simulink model "HILS_Px4"  (Simulink 8.6)
settings: Solver=FixedStepDiscrete  StartTime=0.0  StopTime=inf  FixedStep=0.01  RelTol=1e-3
PreLoadFcn:
  | addpath([cd filesep 'QuadCom']);
InitFcn:
  | %cd('..\Uart_Com');
undefined symbols (not defined in the file or in its folder): DiscIntNeverNeededParam
libraries: vrlib x1, sldrtlib x1
settings Model: Creator=Michael  LastModifiedBy=Xuan Mung  ExtModeTrigDuration=2
settings DataIOCC: SignalLoggingSaveFormat=Dataset
settings OptimizationCC: ExpressionDepthLimit=128  OptimizeModelRefInitCode=on  LifeSpan=1
settings DebuggingCC: SolverPrmCheckMsg=none  FcnCallInpInsideContextMsg=EnableAllAsError  StateNameClashWarn=none
settings HardwareCC: ProdBitPerInt=16  ProdBitPerPointer=8  ProdIntDivRoundTo=Zero  ProdEndianess=LittleEndian  ProdWordSize=8  ProdHWDeviceType=Atmel->AVR
settings RTWCC: SystemTargetFile=realtime.tlc  GenerateMakefile=off  TemplateMakefile=realtime.tmf  Description=Run on Target Hardware  RTWVerbose=off
settings STFCustomTargetCC: TargetLibSuffix=.a  GenerateSampleERTMain=on  ERTCustomFileBanners=on  SupportNonInlinedSFcns=off  SupportVariableSizeSignals=on  MATLABClassNameForMDSCustomization=Simulink.SoftwareTarget.ERTCustomization  GRTInterface=off  SystemTargetFile=realtime.tlc
settings ERTTargetCC: MultiwordLength=2048  GenerateSampleERTMain=on  ParMdlRefBuildCompliant=off  CompOptLevelCompliant=off  ConcurrentExecutionCompliant=off  CombineOutputUpdateFcns=off  ERTFirstTimeCompliant=off  SupportContinuousTime=on  SupportVariableSizeSignals=on  ModelStepFunctionPrototypeControlCompliant=off  CPPClassGenCompliant=off  UseToolchainInfoCompliant=off  ExtModeTransport=3  ExtModeMexFile=ext_serial_win32_comm_rtt  ExtModeMexArgs=0 1 9600  ERTSrcFileBannerTemplate=realtime_code_template.cgt  ERTHdrFileBannerTemplate=realtime_code_template.cgt  ERTDataSrcFileTemplate=realtime_code_template.cgt  ERTDataHdrFileTemplate=realtime_code_template.cgt  ERTCustomFileTemplate=realtime_file_process.tlc  ConvertIfToSwitch=off  SuppressUnreachableDefaultCases=off
settings ConfigComp: CovSFcnEnable=off
settings SettingsController: Description=Run on Hardware Dialog  TargetExtensionPlatform=None
settings MATStruct: Set_host_COM_port=[0.0]  COM_port_number=1  COM_port_baud_rate=115200  Enable_overrun_detection=[0.0]  Digital_output_to_set_on_overrun=13  Extmode_interface_arduino=[0.0]  Analog_input_reference_voltage=[0.0]  Serial0_baud_rate=9600  Serial1_baud_rate=9600  Serial2_baud_rate=9600  Serial3_baud_rate=9600  Local_ip_address=192.168.0.20  Local_mac_address=DE:AD:BE:EF:FE:ED  Wifi_ip_address=192.168.1.20  Wifi_SSID=yourNetwork  Set_Wifi_Encryption=[0.0]  Wifi_WEP_key=D0D0DEADF00DABBADEAFBEADED  Wifi_WEP_key_index=0  Wifi_WPA_password=secretPassword

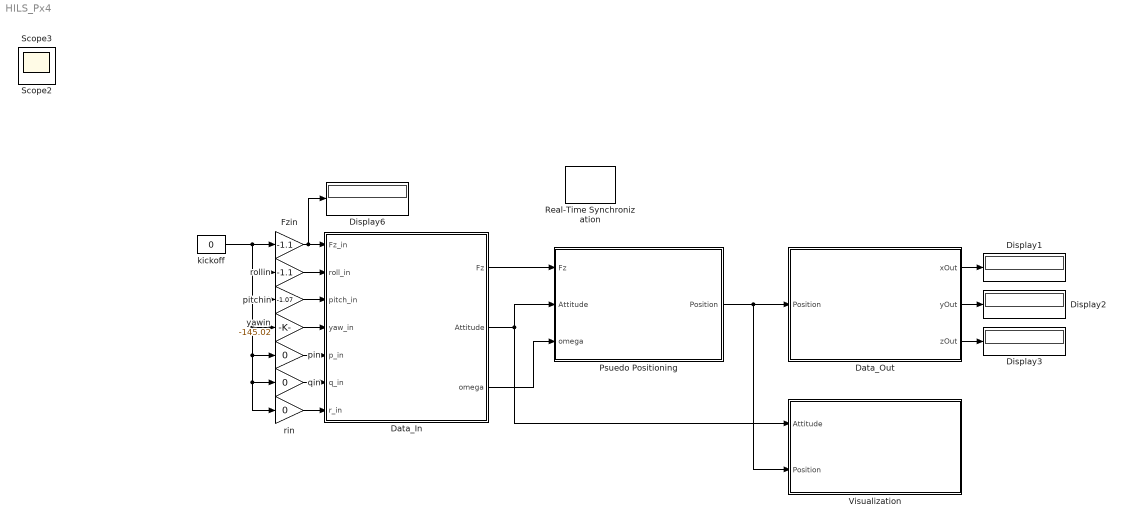
== system HILS_Px4 ==
  Data_In : Subsystem
  Data_Out : Subsystem
  Display{1..3,6} (4 alike) : Display
  Fzin : Gain  Gain=-1.1
  Psuedo Positioning : Subsystem
  Real-Time Synchronization : sldrtlib/Real-Time Synchronization  SampleTime=0.1  MaxMissedTicks=10  ShowMissedTicks=off  YieldWhenWaiting=off
  Visualization : Subsystem
  kickoff : Constant  Value=0
  pin : Gain  Gain=0
  pitchin : Gain  Gain=-1.07
  qin : Gain  Gain=0
  rin : Gain  Gain=0
  rollin : Gain  Gain=-1.1
  yawin : Gain  Gain=-145.02
  Scope2 : Scope
  Scope3 : Scope
  wires:
  Data_Out/1(xOut) -> Display1/1
  Data_Out/2(yOut) -> Display2/1
  Data_Out/3(zOut) -> Display3/1
  Fzin/1 -> Display6/1, Data_In/1(Fz_in)
  rollin/1 -> Data_In/2(roll_in)
  pitchin/1 -> Data_In/3(pitch_in)
  yawin/1 -> Data_In/4(yaw_in)
  pin/1 -> Data_In/5(p_in)
  qin/1 -> Data_In/6(q_in)
  rin/1 -> Data_In/7(r_in)
  kickoff/1 -> pitchin/1, yawin/1, pin/1, qin/1, rin/1, rollin/1, Fzin/1
  Data_In/1(Fz) -> Psuedo Positioning/1(Fz)
  Data_In/2(Attitude) -> Visualization/1(Attitude), Psuedo Positioning/2(Attitude)
  Data_In/3(omega) -> Psuedo Positioning/3(omega)
  Psuedo Positioning/1(Position) -> Visualization/2(Position), Data_Out/1(Position)

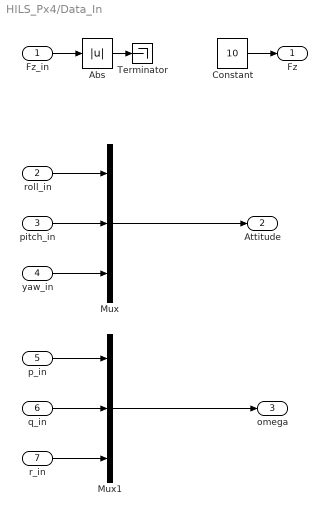
== system HILS_Px4/Data_In ==
  Fz_in : Inport
  roll_in : Inport  Port=2
  pitch_in : Inport  Port=3
  yaw_in : Inport  Port=4
  p_in : Inport  Port=5
  q_in : Inport  Port=6
  r_in : Inport  Port=7
  Abs : Abs
  Constant : Constant  Value=10
  Mux : Mux  Inputs=3
  Mux1 : Mux  Inputs=3
  Terminator : Terminator
  Fz : Outport
  Attitude : Outport  Port=2
  omega : Outport  Port=3
  wires:
  Mux/1 -> Attitude/1
  Mux1/1 -> omega/1
  roll_in/1 -> Mux/1
  pitch_in/1 -> Mux/2
  yaw_in/1 -> Mux/3
  p_in/1 -> Mux1/1
  q_in/1 -> Mux1/2
  r_in/1 -> Mux1/3
  Fz_in/1 -> Abs/1
  Constant/1 -> Fz/1
  Abs/1 -> Terminator/1

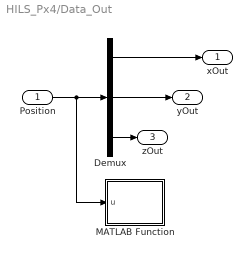
== system HILS_Px4/Data_Out ==
  Position : Inport
  Demux : Demux  Outputs=3
  MATLAB Function : MATLAB Function  TreatAsAtomicUnit=on
  xOut : Outport
  yOut : Outport  Port=2
  zOut : Outport  Port=3
  wires:
  Position/1 -> Demux/1, MATLAB Function/1(u)
  Demux/1 -> xOut/1
  Demux/2 -> yOut/1
  Demux/3 -> zOut/1

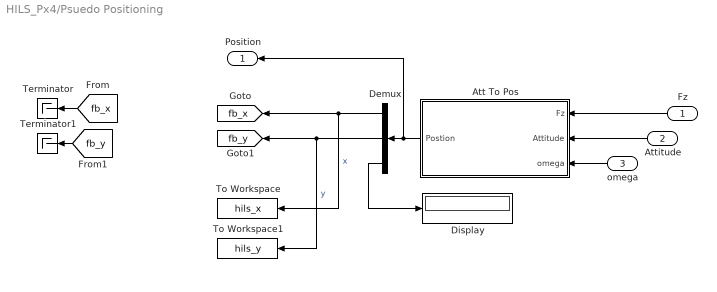
== system HILS_Px4/Psuedo Positioning ==
  Fz : Inport
  Attitude : Inport  Port=2
  omega : Inport  Port=3
  Att To Pos : Subsystem
  Demux : Demux  Outputs=3
  Display : Display
  Terminator : Terminator
  Terminator1 : Terminator
  To Workspace : ToWorkspace  VariableName=hils_x  SaveFormat=Timeseries  SampleTime=-1
  To Workspace1 : ToWorkspace  VariableName=hils_y  SaveFormat=Timeseries  SampleTime=-1
  Position : Outport
  tag scope: fb_x=global, fb_y=global
  wires:
  Attitude/1 -> Att To Pos/2(Attitude)
  Att To Pos/1(Postion) -> Position/1, Demux/1
  Demux/1 -> [fb_x], To Workspace/1  "x"
  Demux/2 -> [fb_y], To Workspace1/1  "y"
  omega/1 -> Att To Pos/3(omega)
  Demux/3 -> Display/1
  Fz/1 -> Att To Pos/1(Fz)
  [fb_x] -> Terminator/1
  [fb_y] -> Terminator1/1

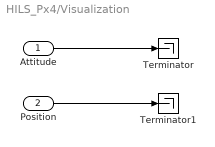
== system HILS_Px4/Visualization ==
  Attitude : Inport
  Position : Inport  Port=2
  Terminator : Terminator
  Terminator1 : Terminator
  wires:
  Attitude/1 -> Terminator/1
  Position/1 -> Terminator1/1

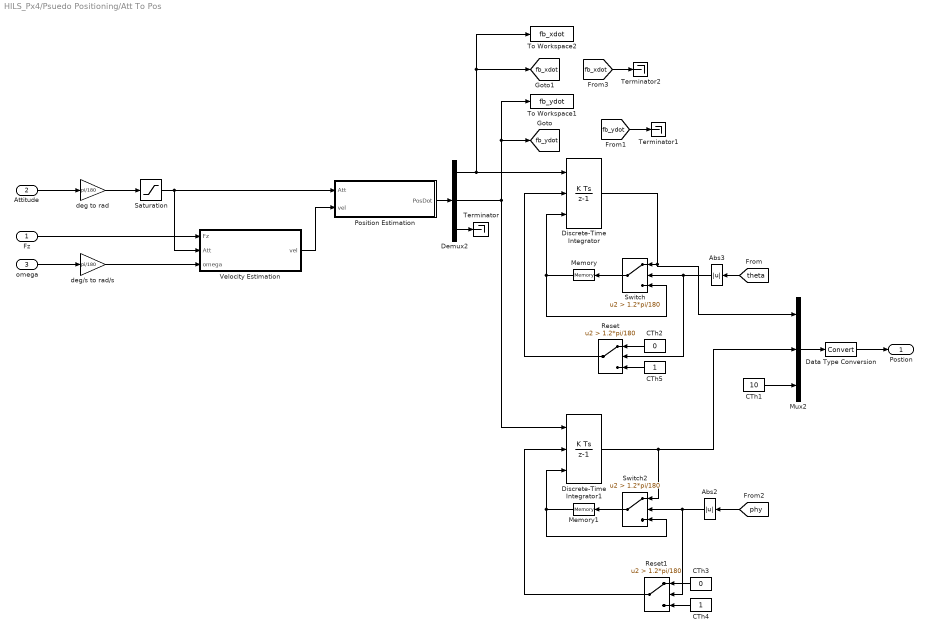
== system HILS_Px4/Psuedo Positioning/Att To Pos ==
  Fz : Inport
  Attitude : Inport  Port=2
  omega : Inport  Port=3
  Abs2 : Abs
  Abs3 : Abs
  CTh1 : Constant  Value=10
  CTh2 : Constant  Value=0
  CTh3 : Constant  Value=0
  CTh4 : Constant
  CTh5 : Constant
  Data Type Conversion : DataTypeConversion
  Demux2 : Demux  Outputs=3
  Discrete-Time Integrator : DiscreteIntegrator  gainval=1  ExternalReset=level  InitialConditionSource=external  InitialConditionSetting=State (most efficient)  SampleTime=-1  ICPrevOutput=DiscIntNeverNeededParam  ICPrevScaledInput=DiscIntNeverNeededParam
  Discrete-Time Integrator1 : DiscreteIntegrator  gainval=1  ExternalReset=level  InitialConditionSource=external  InitialConditionSetting=State (most efficient)  SampleTime=-1  ICPrevOutput=DiscIntNeverNeededParam  ICPrevScaledInput=DiscIntNeverNeededParam
  Memory : Memory
  Memory1 : Memory
  Mux2 : Mux  Inputs=3
  Position Estimation : Subsystem
  Reset : Switch  Criteria=u2 > Threshold  Threshold=1.2*pi/180
  Reset1 : Switch  Criteria=u2 > Threshold  Threshold=1.2*pi/180
  Saturation : Saturate  UpperLimit=1.99*pi  LowerLimit=-1.99*pi
  Switch : Switch  Criteria=u2 > Threshold  Threshold=1.2*pi/180
  Switch2 : Switch  Criteria=u2 > Threshold  Threshold=1.2*pi/180
  Terminator : Terminator
  Terminator1 : Terminator
  Terminator2 : Terminator
  To Workspace1 : ToWorkspace  VariableName=fb_ydot  SaveFormat=Timeseries  SampleTime=-1
  To Workspace2 : ToWorkspace  VariableName=fb_xdot  SaveFormat=Timeseries  SampleTime=-1
  Velocity Estimation : Subsystem
  deg to rad : Gain  Gain=pi/180  OutDataTypeStr=Inherit: Same as input
  deg/s to rad/s : Gain  Gain=pi/180  OutDataTypeStr=Inherit: Same as input
  Postion : Outport
  tag scope: fb_xdot=global, fb_ydot=global
  wires:
  Velocity Estimation/1(vel) -> Position Estimation/2(vel)
  omega/1 -> deg/s to rad/s/1
  deg to rad/1 -> Saturation/1
  Fz/1 -> Velocity Estimation/1(Fz)
  Attitude/1 -> deg to rad/1
  Position Estimation/1(PosDot) -> Demux2/1
  deg/s to rad/s/1 -> Velocity Estimation/3(omega)
  Memory/1 -> Switch/3, Discrete-Time Integrator/3
  Abs3/1 -> Reset/2, Switch/2
  [theta] -> Abs3/1
  Discrete-Time Integrator/1 -> Mux2/1, Switch/1
  Switch/1 -> Memory/1
  Demux2/1 -> To Workspace2/1, [fb_xdot], Discrete-Time Integrator/1
  Data Type Conversion/1 -> Postion/1
  Mux2/1 -> Data Type Conversion/1
  Memory1/1 -> Switch2/3, Discrete-Time Integrator1/3
  Abs2/1 -> Reset1/2, Switch2/2
  [phy] -> Abs2/1
  Discrete-Time Integrator1/1 -> Mux2/2, Switch2/1
  Switch2/1 -> Memory1/1
  Demux2/2 -> Discrete-Time Integrator1/1, To Workspace1/1, [fb_ydot]
  CTh2/1 -> Reset/1
  CTh5/1 -> Reset/3
  Reset/1 -> Discrete-Time Integrator/2
  CTh3/1 -> Reset1/1
  CTh4/1 -> Reset1/3
  Reset1/1 -> Discrete-Time Integrator1/2
  CTh1/1 -> Mux2/3
  Demux2/3 -> Terminator/1
  Saturation/1 -> Velocity Estimation/2(Att), Position Estimation/1(Att)
  [fb_ydot] -> Terminator1/1
  [fb_xdot] -> Terminator2/1

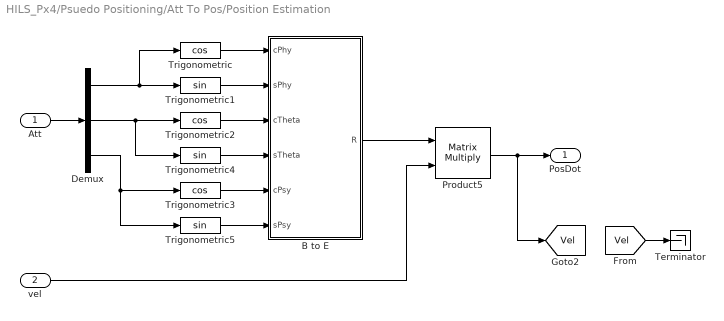
== system HILS_Px4/Psuedo Positioning/Att To Pos/Position Estimation ==
  Att : Inport
  vel : Inport  Port=2
  B to E : MATLAB Function  TreatAsAtomicUnit=on
  Demux : Demux  Outputs=3
  Product5 : Product  Multiplication=Matrix(*)
  Terminator : Terminator
  Trigonometric : Trigonometry  Operator=cos  NumberOfIterations=32
  Trigonometric1 : Trigonometry  NumberOfIterations=32
  Trigonometric2 : Trigonometry  Operator=cos  NumberOfIterations=32
  Trigonometric3 : Trigonometry  Operator=cos  NumberOfIterations=32
  Trigonometric4 : Trigonometry  NumberOfIterations=32
  Trigonometric5 : Trigonometry  NumberOfIterations=32
  PosDot : Outport
  tag scope: Vel=global
  wires:
  Demux/1 -> Trigonometric1/1, Trigonometric/1
  Demux/2 -> Trigonometric4/1, Trigonometric2/1
  Trigonometric/1 -> B to E/1(cPhy)
  Trigonometric1/1 -> B to E/2(sPhy)
  Trigonometric2/1 -> B to E/3(cTheta)
  Trigonometric4/1 -> B to E/4(sTheta)
  Trigonometric3/1 -> B to E/5(cPsy)
  Trigonometric5/1 -> B to E/6(sPsy)
  B to E/1(R) -> Product5/1
  vel/1 -> Product5/2
  Demux/3 -> Trigonometric5/1, Trigonometric3/1
  Att/1 -> Demux/1
  Product5/1 -> [Vel], PosDot/1
  [Vel] -> Terminator/1

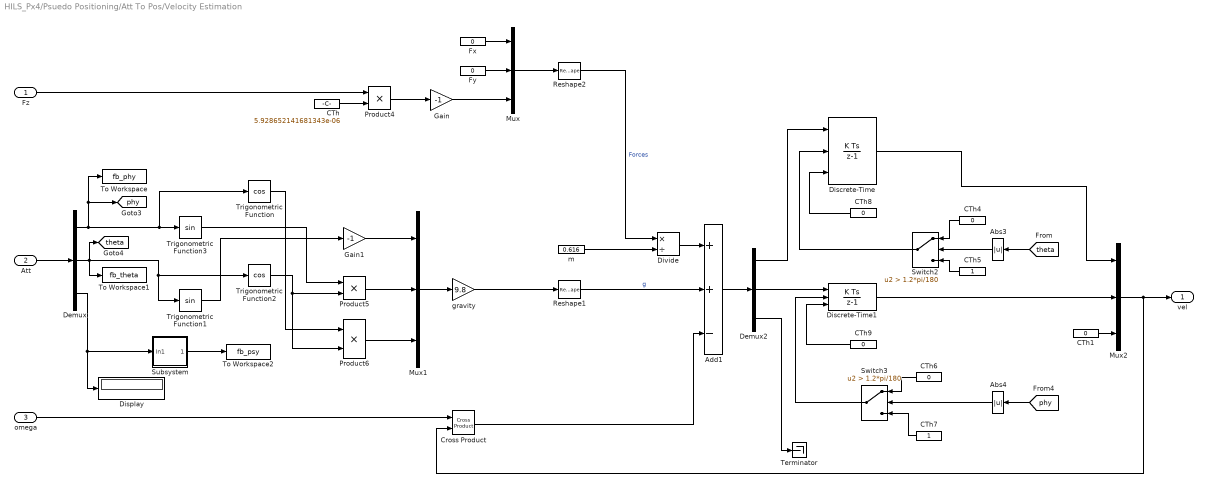
== system HILS_Px4/Psuedo Positioning/Att To Pos/Velocity Estimation ==
  Fz : Inport
  Att : Inport  Port=2
  omega : Inport  Port=3
  Abs3 : Abs
  Abs4 : Abs
  Add1 : Sum  Inputs=++-
  CTh : Constant  Value=5.928652141681343e-06
  CTh{1,4,6,8..9} (5 alike) : Constant  Value=0
  CTh5 : Constant
  CTh7 : Constant
  Cross Product : vrlib/Utilities/Cross Product
  Demux : Demux  Outputs=3
  Demux2 : Demux  Outputs=3
  Discrete-Time : DiscreteIntegrator  gainval=1  ExternalReset=level  InitialConditionSource=external  InitialConditionSetting=State (most efficient)  SampleTime=-1  ICPrevOutput=DiscIntNeverNeededParam  ICPrevScaledInput=DiscIntNeverNeededParam
  Discrete-Time1 : DiscreteIntegrator  gainval=1  ExternalReset=level  InitialConditionSource=external  InitialConditionSetting=State (most efficient)  SampleTime=-1  ICPrevOutput=DiscIntNeverNeededParam  ICPrevScaledInput=DiscIntNeverNeededParam
  Display : Display
  Divide : Product  Inputs=*/
  Fx : Constant  Value=0
  Fy : Constant  Value=0
  Gain : Gain  Gain=-1
  Gain1 : Gain  Gain=-1
  Mux : Mux  Inputs=3
  Mux1 : Mux  Inputs=3
  Mux2 : Mux  Inputs=3
  Product4 : Product
  Product5 : Product
  Product6 : Product
  Reshape1 : Reshape  OutputDimensionality=Column vector (2-D)
  Reshape2 : Reshape  OutputDimensionality=Column vector (2-D)
  Subsystem : Subsystem
  Switch2 : Switch  Criteria=u2 > Threshold  Threshold=1.2*pi/180
  Switch3 : Switch  Criteria=u2 > Threshold  Threshold=1.2*pi/180
  Terminator : Terminator
  To Workspace : ToWorkspace  VariableName=fb_phy  SaveFormat=Timeseries  SampleTime=-1
  To Workspace1 : ToWorkspace  VariableName=fb_theta  SaveFormat=Timeseries  SampleTime=-1
  To Workspace2 : ToWorkspace  VariableName=fb_psy  SaveFormat=Timeseries  SampleTime=-1
  Trigonometric Function : Trigonometry  Operator=cos  NumberOfIterations=32
  Trigonometric Function1 : Trigonometry  NumberOfIterations=32
  Trigonometric Function2 : Trigonometry  Operator=cos  NumberOfIterations=32
  Trigonometric Function3 : Trigonometry  NumberOfIterations=32
  gravity : Gain  Gain=9.8
  m : Constant  Value=0.616
  vel : Outport
  tag scope: phy=global, theta=global
  wires:
  Fz/1 -> Product4/1
  CTh/1 -> Product4/2
  Product4/1 -> Gain/1
  Gain/1 -> Mux/3
  Fy/1 -> Mux/2
  Fx/1 -> Mux/1
  Demux/1 -> To Workspace/1, [phy], Trigonometric Function/1, Trigonometric Function3/1
  Demux/2 -> To Workspace1/1, [theta], Trigonometric Function1/1, Trigonometric Function2/1
  Mux1/1 -> gravity/1
  Gain1/1 -> Mux1/1
  Trigonometric Function1/1 -> Gain1/1
  Trigonometric Function3/1 -> Product5/1
  Trigonometric Function2/1 -> Product6/2, Product5/2
  Product5/1 -> Mux1/2
  Trigonometric Function/1 -> Product6/1
  Product6/1 -> Mux1/3
  m/1 -> Divide/2
  Mux/1 -> Reshape2/1
  Reshape1/1 -> Add1/2  "g"
  Cross Product/1 -> Add1/3
  Att/1 -> Demux/1
  omega/1 -> Cross Product/1
  Demux/3 -> Subsystem/1(In1), Display/1
  Divide/1 -> Add1/1
  Reshape2/1 -> Divide/1  "Forces"
  gravity/1 -> Reshape1/1
  Add1/1 -> Demux2/1
  Demux2/1 -> Discrete-Time/1
  Discrete-Time/1 -> Mux2/1
  CTh8/1 -> Discrete-Time/3
  Demux2/2 -> Discrete-Time1/1
  Demux2/3 -> Terminator/1
  Mux2/1 -> Cross Product/2, vel/1
  Abs3/1 -> Switch2/2
  [theta] -> Abs3/1
  Discrete-Time1/1 -> Mux2/2
  CTh9/1 -> Discrete-Time1/3
  Abs4/1 -> Switch3/2
  [phy] -> Abs4/1
  CTh1/1 -> Mux2/3
  CTh5/1 -> Switch2/3
  CTh4/1 -> Switch2/1
  Switch2/1 -> Discrete-Time/2
  CTh7/1 -> Switch3/3
  CTh6/1 -> Switch3/1
  Switch3/1 -> Discrete-Time1/2
  Subsystem/1(Out1) -> To Workspace2/1

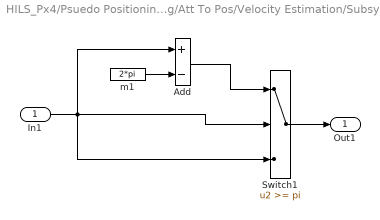
== system HILS_Px4/Psuedo Positioning/Att To Pos/Velocity Estimation/Subsystem ==
  In1 : Inport
  Add : Sum  Inputs=+-
  Switch1 : Switch  Threshold=pi
  m1 : Constant  Value=2*pi
  Out1 : Outport
  wires:
  Switch1/1 -> Out1/1
  m1/1 -> Add/2
  In1/1 -> Add/1, Switch1/2, Switch1/3
  Add/1 -> Switch1/1

== matlab function Psuedo Positioning/Att To Pos/Position Estimation/B to E ==
  data: cPhy input double; sPhy input double; cTheta input double; sTheta input double; cPsy input double; sPsy input double; R output double
function R = fcn(cPhy, sPhy, cTheta, sTheta, cPsy, sPsy)
%#codegen
% phi = attitude(1);
% theta = attitude(2);
% psi = attitude(3);

% Calculate the rotational Matrix
R = [cTheta*cPsy  sPhy*sTheta*cPsy-cPhy*sPsy  cPhy*sTheta*cPsy+sPhy*sPsy;...
     cTheta*sPsy  sPhy*sTheta*sPsy+cPhy*cPsy  cPhy*sTheta*sPsy-sPhy*cPsy;...
     -sTheta              sPhy*cTheta                      cPhy*cTheta];

%  R = fxdt(R,1,32,16);

%  posDot = R*vel;

== matlab function Data_Out/MATLAB Function ==
  data: u input double
function fcn(u)
coder.extrinsic('set_param'); 
% set_param('HILS_Px4/Out', 'UserData', u);
set_param('HILS_Px4/Data_Out/xOut', 'UserData', u(1));
set_param('HILS_Px4/Data_Out/yOut', 'UserData', u(2));
set_param('HILS_Px4/Data_Out/zOut', 'UserData', u(3));
end
